simulink model "NonlinearModel1"  (R2015a)
settings: Solver=ode45  StartTime=0.0  StopTime=10.0  RelTol=1e-3
values from neighbouring files (symbols this model uses):
  Fg = 9.82 * m    (= 4.91)    [Parameters.m]
  Jx = 0.2    [Parameters.m]
  Jy = 0.2    [Parameters.m]
  Jz = 0.4    [Parameters.m]
  kd = 0.0001    [Parameters.m]
  kth = 0.04    [Parameters.m]
  L = 0.16    [Parameters.m]
  m = 0.5    [Parameters.m]
libraries: simulink x4
settings Model: Creator=Amalie  LastModifiedBy=Amalie

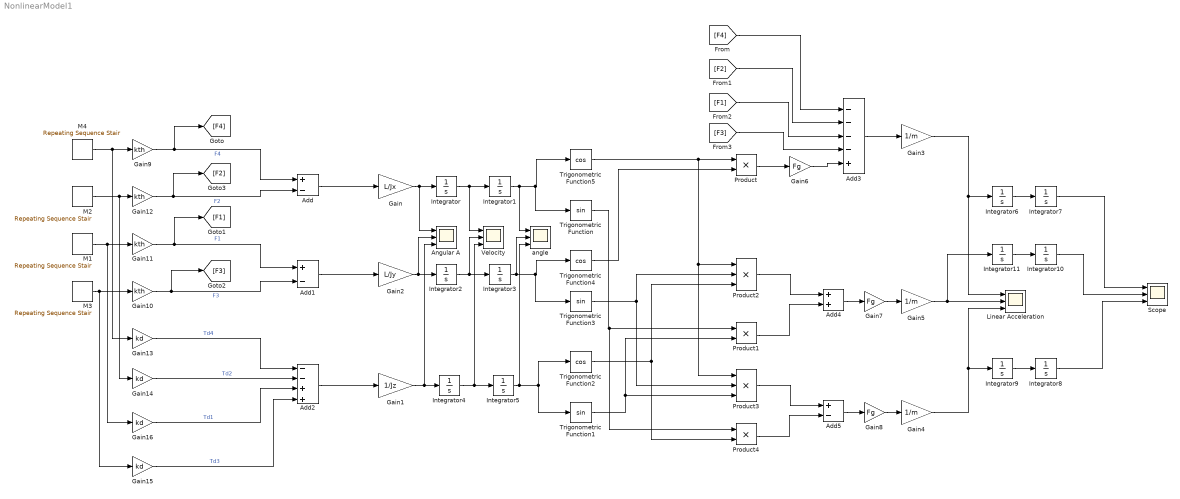
== system NonlinearModel1 ==
  Add : Sum  Inputs=+-
  Add1 : Sum  Inputs=+-
  Add2 : Sum  Inputs=--++
  Add3 : Sum  Inputs=----+
  Add4 : Sum
  Add5 : Sum  Inputs=+-
  Angular A : Scope  NumInputPorts=3
      settings: YMin=-5~-5~-5  YMax=5~5~5  SaveName=ScopeData3
  Gain : Gain  Gain=L/Jx
  Gain1 : Gain  Gain=1/Jz
  Gain{9..12} (4 alike) : Gain  Gain=kth
  Gain{13..16} (4 alike) : Gain  Gain=kd
  Gain2 : Gain  Gain=L/Jy
  Gain3 : Gain  Gain=1/m
  Gain4 : Gain  Gain=1/m
  Gain5 : Gain  Gain=1/m
  Gain6 : Gain  Gain=Fg
  Gain7 : Gain  Gain=Fg
  Gain8 : Gain  Gain=Fg
  Integrator{,1..11} (12 alike) : Integrator
  Linear Acceleration : Scope  NumInputPorts=3
      settings: YMin=-5~-5~-5  YMax=5~5~5
  M1 : simulink/Sources/Repeating Sequence Stair  OutValues=[30].'  tsamp=0.1  OutMin=[]  OutMax=[]  OutDataTypeStr=double  OutputDataTypeScalingMode=double  OutDataType=fixdt(0,8)  ConRadixGroup=Best Precision: Vector-wise  OutScaling=2^-12
  M2 : simulink/Sources/Repeating Sequence Stair  OutValues=[30 40 30 20 30 20 30 40].'  tsamp=0.5  OutMin=[]  OutMax=[]  OutDataTypeStr=double  OutputDataTypeScalingMode=double  OutDataType=fixdt(0,8)  ConRadixGroup=Best Precision: Vector-wise  OutScaling=2^-12
  M3 : simulink/Sources/Repeating Sequence Stair  OutValues=[30].'  tsamp=0.1  OutMin=[]  OutMax=[]  OutDataTypeStr=double  OutputDataTypeScalingMode=double  OutDataType=fixdt(0,8)  ConRadixGroup=Best Precision: Vector-wise  OutScaling=2^-12
  M4 : simulink/Sources/Repeating Sequence Stair  OutValues=[30 20 30 40 30 40 30 20].'  tsamp=0.5  OutMin=[]  OutMax=[]  OutDataTypeStr=double  OutputDataTypeScalingMode=double  OutDataType=fixdt(0,8)  ConRadixGroup=Best Precision: Vector-wise  OutScaling=2^-12
  Product : Product
  Product1 : Product
  Product2 : Product  Inputs=3
  Product3 : Product  Inputs=3
  Product4 : Product
  Scope : Scope  NumInputPorts=3
      settings: YMin=-5~-5~-5  YMax=5~5~5  SaveName=ScopeData4
  Trigonometric Function : Trigonometry
  Trigonometric Function1 : Trigonometry
  Trigonometric Function2 : Trigonometry  Operator=cos
  Trigonometric Function3 : Trigonometry
  Trigonometric Function4 : Trigonometry  Operator=cos
  Trigonometric Function5 : Trigonometry  Operator=cos
  Velocity : Scope  NumInputPorts=3
      settings: YMin=-5~-5~-5  YMax=5~5~5  SaveName=ScopeData2
  angle : Scope  NumInputPorts=3
      settings: YMin=-5~-5~-5  YMax=5~5~5
  wires:
  Add2/1 -> Gain1/1
  Add1/1 -> Gain2/1
  Add/1 -> Gain/1
  Gain/1 -> Angular A/1, Integrator/1
  Gain2/1 -> Angular A/2, Integrator2/1
  Gain1/1 -> Angular A/3, Integrator4/1
  Integrator4/1 -> Velocity/3, Integrator5/1
  Integrator2/1 -> Velocity/2, Integrator3/1
  Integrator/1 -> Velocity/1, Integrator1/1
  Integrator1/1 -> angle/1, Trigonometric Function/1, Trigonometric Function5/1
  Integrator3/1 -> angle/2, Trigonometric Function3/1, Trigonometric Function4/1
  Integrator5/1 -> Trigonometric Function1/1, Trigonometric Function2/1, angle/3
  Trigonometric Function5/1 -> Product2/1, Product3/1, Product/1
  Trigonometric Function4/1 -> Product/2
  Trigonometric Function3/1 -> Product2/2, Product3/2
  Trigonometric Function2/1 -> Product2/3, Product4/2
  Trigonometric Function/1 -> Product4/1, Product1/1
  Trigonometric Function1/1 -> Product3/3, Product1/2
  Product/1 -> Gain6/1
  Product2/1 -> Add4/1
  Product1/1 -> Add4/2
  Product3/1 -> Add5/1
  Product4/1 -> Add5/2
  Add3/1 -> Gain3/1
  Add4/1 -> Gain7/1
  Add5/1 -> Gain8/1
  Gain7/1 -> Gain5/1
  Gain8/1 -> Gain4/1
  M4/1 -> Gain13/1, Gain9/1
  M2/1 -> Gain14/1, Gain12/1
  M1/1 -> Gain16/1, Gain11/1
  M3/1 -> Gain15/1, Gain10/1
  Gain9/1 -> [F4], Add/1  "F4"
  Gain12/1 -> [F2], Add/2  "F2"
  Gain10/1 -> Add1/2, [F3]  "F3"
  Gain11/1 -> [F1], Add1/1  "F1"
  Gain14/1 -> Add2/2  "Td2"
  Gain13/1 -> Add2/1  "Td4"
  Gain16/1 -> Add2/3  "Td1"
  Gain15/1 -> Add2/4  "Td3"
  [F4] -> Add3/1
  [F2] -> Add3/2
  [F1] -> Add3/3
  [F3] -> Add3/4
  Gain6/1 -> Add3/5
  Gain3/1 -> Integrator6/1, Linear Acceleration/1
  Gain5/1 -> Integrator11/1, Linear Acceleration/2
  Gain4/1 -> Integrator9/1, Linear Acceleration/3
  Integrator6/1 -> Integrator7/1
  Integrator9/1 -> Integrator8/1
  Integrator11/1 -> Integrator10/1
  Integrator7/1 -> Scope/1
  Integrator10/1 -> Scope/2
  Integrator8/1 -> Scope/3
